simulink model "Final_Design_Updated"  (R2017b)
settings: Solver=VariableStepAuto  StartTime=0.0  StopTime=250  RelTol=1e-3
libraries: xbsIndex_r4 x101
settings Model: Creator=the20  LastModifiedBy=the20

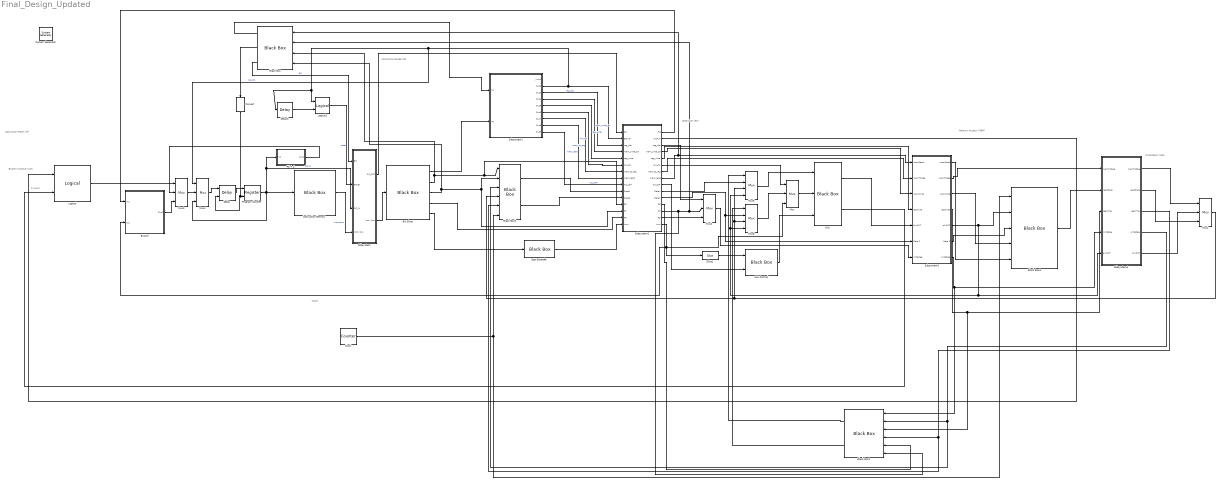
== system Final_Design_Updated ==
  note: Write Back (WB)
  note: Memory Access (MEM)
  note: Execution (EX)
  note: Instruction Dcode (ID)
  note: Branch (Control Unit)
  note: Z (ALU)
  note: Clock
  note: Instruction Fetch (IF)
  " System Generator" : xbsIndex_r4/ System Generator  Tag=genX  xilinxfamily=kintex7  part=xc7k325t  speed=-3  package=fbg676  synthesis_tool=Vivado  clock_wrapper=Clock Enables  directory=./netlist  proj_type=Vivado  Synth_file=Vivado Synthesis Defaults  Impl_file=Vivado Implementation Defaults  testbench=off  simulink_period=1  sysclk_period=10  dcm_input_clock_period=10  incr_netlist=off  trim_vbits=Everywhere in SubSystem  dbl_ovrd=According to Block Masks  core_generation=According to Block Masks  run_coregen=off  deprecated_control=off  eval_field=0  block_type=sysgen
  ALU : xbsIndex_r4/Black Box  init_code=mipsalu_config  sim_method=ISE Simulator  verbose=off  block_type=blackbox2
  ALU Control : xbsIndex_r4/Black Box  init_code=ALU_Control_config  sim_method=ISE Simulator  verbose=off  block_type=blackbox2
  Bit Slicer : xbsIndex_r4/Black Box  init_code=Bit_Slicer_config  sim_method=ISE Simulator  verbose=off  block_type=blackbox2
  Black Box : xbsIndex_r4/Black Box  init_code=Hazard_Unit_config  sim_method=ISE Simulator  verbose=off  block_type=blackbox2
  Black Box1 : xbsIndex_r4/Black Box  init_code=Forwarding_Unit_config  sim_method=ISE Simulator  verbose=off  block_type=blackbox2
  Black Box2 : xbsIndex_r4/Black Box  init_code=regFile_config  sim_method=ISE Simulator  verbose=off  block_type=blackbox2
  Black Box3 : xbsIndex_r4/Black Box  init_code=Data_Memory_config  sim_method=ISE Simulator  verbose=off  block_type=blackbox2
  Branch : Subsystem
  Clock : xbsIndex_r4/Counter  cnt_type=Free Running  cnt_to=Inf  operation=Up  start_count=0  cnt_by_val=1  arith_type=Unsigned  n_bits=1  bin_pt=0  load_pin=off  rst=off  en=off  explicit_period=on  period=1  use_behavioral_HDL=off  implementation=Fabric  dbl_ovrd=off  block_type=counter
  Convert : xbsIndex_r4/Convert  gui_display_data_type=Boolean  arith_type=Boolean  n_bits=16  bin_pt=14  float_type=Single  exp_bits=8  fraction_bits=24  quantization=Truncate  overflow=Wrap  en=off  latency=0  pipeline=off  dbl_ovrd=off  block_type=convert
  "Delay " : xbsIndex_r4/Delay  rst=off  infoeditControl=Selection of Reset will increase slice count due to use of real FFs and instead of SRLs  en=on  latency=1  reg_retiming=off  dbl_ovrd=off  block_type=delay
  Delay3 : xbsIndex_r4/Delay  rst=off  infoeditControl=Selection of Reset will increase slice count due to use of real FFs and instead of SRLs  en=off  latency=1  reg_retiming=off  dbl_ovrd=off  block_type=delay
  Instruction Memory : xbsIndex_r4/Black Box  init_code=InstructionMemory_config  sim_method=ISE Simulator  verbose=off  block_type=blackbox2
  Logical : xbsIndex_r4/Logical  logical_function=AND  inputs=2  en=off  latency=0  precision=Full  arith_type=Unsigned  n_bits=16  bin_pt=0  align_bp=on  dbl_ovrd=off  block_type=logical
  Logical1 : xbsIndex_r4/Logical  logical_function=OR  inputs=2  en=off  latency=1  precision=Full  arith_type=Unsigned  n_bits=16  bin_pt=0  align_bp=on  dbl_ovrd=off  block_type=logical
  Mux : xbsIndex_r4/Mux  inputs=2  en=off  latency=0  precision=Full  arith_type=Unsigned  n_bits=16  bin_pt=14  quantization=Truncate  overflow=Wrap  dbl_ovrd=off  block_type=mux
  Mux1 : xbsIndex_r4/Mux  inputs=2  en=off  latency=0  precision=Full  arith_type=Unsigned  n_bits=16  bin_pt=14  quantization=Truncate  overflow=Wrap  dbl_ovrd=off  block_type=mux
  Mux2 : xbsIndex_r4/Mux  inputs=2  en=off  latency=0  precision=Full  arith_type=Unsigned  n_bits=16  bin_pt=14  quantization=Truncate  overflow=Wrap  dbl_ovrd=off  block_type=mux
  Mux3 : xbsIndex_r4/Mux  inputs=2  en=off  latency=0  precision=User Defined  arith_type=Unsigned  n_bits=32  bin_pt=0  quantization=Truncate  overflow=Wrap  dbl_ovrd=off  block_type=mux
  Mux4 : xbsIndex_r4/Mux  inputs=2  en=off  latency=0  precision=User Defined  arith_type=Unsigned  n_bits=32  bin_pt=0  quantization=Truncate  overflow=Wrap  dbl_ovrd=off  block_type=mux
  Mux5 : xbsIndex_r4/Mux  inputs=3  en=off  latency=0  precision=Full  arith_type=Unsigned  n_bits=16  bin_pt=14  quantization=Truncate  overflow=Wrap  dbl_ovrd=off  block_type=mux
  Mux6 : xbsIndex_r4/Mux  inputs=3  en=off  latency=0  precision=Full  arith_type=Unsigned  n_bits=16  bin_pt=14  quantization=Truncate  overflow=Wrap  dbl_ovrd=off  block_type=mux
  PC + 4 : Subsystem
  "Program Counter " : xbsIndex_r4/Register  init=0  rst=off  en=on  dbl_ovrd=off  block_type=register
  Sign Extender : xbsIndex_r4/Black Box  init_code=Sign_Extender_config  sim_method=ISE Simulator  verbose=off  block_type=blackbox2
  Slice1 : xbsIndex_r4/Slice  nbits=6  boolean_output=off  mode=Lower Bit Location + Width  bit1=0  base1=MSB of Input  bit0=0  base0=LSB of Input  dbl_ovrd=off  block_type=slice
  Subsystem : Subsystem
  Subsystem1 : Subsystem
  Subsystem2 : Subsystem
  Subsystem3 : Subsystem
  Subsystem4 : Subsystem
  wires:
  Bit Slicer/5 -> Sign Extender/1
  Mux/1 -> ALU/2
  Mux1/1 -> Black Box2/4, Mux5/3, Mux6/3
  ALU Control/1 -> ALU/3
  Clock/1 -> Black Box3/1, Black Box2/6
  Logical/1 -> Mux3/1
  ALU/2 -> Logical/2
  "Program Counter "/1 -> PC + 4/1(In1), Subsystem/3("PC_IN "), Mux4/3, Instruction Memory/1  "PC_IN"
  Branch/1(Out1) -> Mux3/3
  PC + 4/1(Out1) -> Mux3/2
  Mux3/1 -> Mux4/2
  "Delay "/1 -> "Program Counter "/1
  Mux4/1 -> "Delay "/1
  Delay3/1 -> Logical1/2
  Black Box/2 -> Convert/1
  Black Box/3 -> Subsystem/1(EN)  "EN"
  Logical1/1 -> Subsystem/2("Reset ")  "reset"
  Instruction Memory/1 -> Subsystem/4("Instruction ")  "Instruction"
  Subsystem/2(Instruction) -> Bit Slicer/1
  Subsystem1/2(Out2) -> Subsystem2/2(Branch), Mux4/1, Delay3/1, Logical1/1  "branch"
  Bit Slicer/1 -> Subsystem1/2(In2)
  Convert/1 -> "Delay "/2, "Program Counter "/2
  Black Box/1 -> Subsystem1/1(In1)
  Subsystem/1(PC_OUT) -> Subsystem2/1("PC ")
  Subsystem2/2(branch) -> Logical/1
  Subsystem1/3(Out3) -> Subsystem2/3(reg_dst)  "reg_dst"
  Subsystem1/4(Out4) -> Subsystem2/4(mem_write_en)  "mem_write_en"
  Subsystem1/5(Out5) -> Subsystem2/5(reg_write)  "reg_write"
  Subsystem1/6(Out6) -> Subsystem2/6(Alu_src)  "Alu_src"
  Subsystem1/7(Out7) -> Subsystem2/7(mem_to_reg)  "mem_to_reg"
  Subsystem1/8(Out8) -> Subsystem2/8(mem_read)  "mem_read"
  Subsystem1/9(Out9) -> Subsystem2/9(ALU_OP)  "ALU_OP"
  Black Box2/1 -> Subsystem2/10(Data1)
  Black Box2/2 -> Subsystem2/11(Data2)
  Bit Slicer/4 -> Subsystem2/14(RD)
  Sign Extender/1 -> Subsystem2/15(Imm)
  Bit Slicer/2 -> Black Box/3, Black Box2/1, Subsystem2/12(RS)
  Bit Slicer/3 -> Black Box/4, Black Box2/2, Subsystem2/13(RT)
  Subsystem2/1(PC) -> Branch/1(In1)
  Subsystem2/3("reg_dst ") -> Mux2/1
  Subsystem2/14("RD ") -> Mux2/3
  Subsystem2/6("Alu_src ") -> Mux/1
  Subsystem2/9("ALU_OP ") -> ALU Control/2
  Mux5/1 -> ALU/1
  Mux6/1 -> Mux/2
  Subsystem2/10("Data1 ") -> Mux5/2
  Subsystem2/11("Data2 ") -> Subsystem3/6(Data 2), Mux6/2
  Subsystem2/8("mem_read ") -> Black Box/1, Subsystem3/1("memRead ")
  Subsystem2/7("mem_to_reg ") -> Subsystem3/2(memToReg)
  Subsystem2/4("mem_write_en ") -> Subsystem3/3(memWrite)
  Subsystem2/5("reg_write ") -> Subsystem3/4(regWrite)
  ALU/1 -> Subsystem3/5(aluOUT)
  Mux2/1 -> Subsystem3/7(writeReg)
  Subsystem3/1("memRead ") -> Black Box3/5
  Subsystem3/2("memToReg ") -> Subsystem4/1("memToReg ")
  Black Box3/1 -> Subsystem4/2(readData)
  Subsystem3/4("regWrite ") -> Black Box1/3, Subsystem4/3(regWrite)
  Subsystem3/7("writeReg ") -> Black Box1/1, Subsystem4/4(writeReg)
  Subsystem3/5("aluOUT ") -> Black Box3/2, Mux5/4, Mux6/4, Subsystem4/5(aluOUT)
  Subsystem3/6("Data 2 ") -> Black Box3/3
  Subsystem3/3("memWrite ") -> Black Box3/4
  Subsystem4/1("memToReg ") -> Mux1/1
  Subsystem4/2("readData ") -> Mux1/3
  Subsystem4/5("aluOUT ") -> Mux1/2
  Subsystem4/3("regWrite ") -> Black Box1/4, Black Box2/5
  Subsystem4/4("writeReg ") -> Black Box1/2, Black Box2/3
  Slice1/1 -> ALU Control/1
  Subsystem2/15("Imm ") -> Branch/2(In2), Mux/3, Slice1/1
  Black Box1/1 -> Mux5/1
  Black Box1/2 -> Mux6/1
  Subsystem2/12("RS ") -> Black Box1/5
  Subsystem2/13("RT ") -> Black Box1/6, Black Box/2, Mux2/2

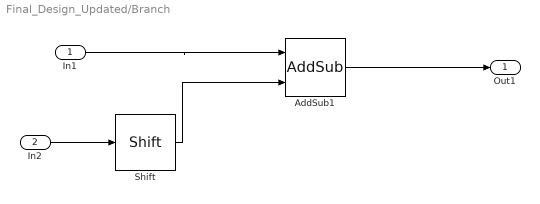
== system Final_Design_Updated/Branch ==
  In1 : Inport
  In2 : Inport  Port=2
  AddSub1 : xbsIndex_r4/AddSub  mode=Addition  use_carryin=off  use_carryout=off  en=off  latency=0  precision=User Defined  arith_type="Signed  (2's comp)"  n_bits=32  bin_pt=0  quantization=Truncate  overflow=Wrap  use_behavioral_HDL=off  hw_selection=Fabric  pipelined=off  dbl_ovrd=off  block_type=addsub
  Shift : xbsIndex_r4/Shift  shift_dir=Left  shift_bits=2  en=off  latency=0  precision=User Defined  arith_type=Unsigned  n_bits=32  bin_pt=0  quantization=Truncate  overflow=Wrap  dbl_ovrd=off  block_type=shift
  Out1 : Outport
  wires:
  AddSub1/1 -> Out1/1
  Shift/1 -> AddSub1/2
  In2/1 -> Shift/1
  In1/1 -> AddSub1/1

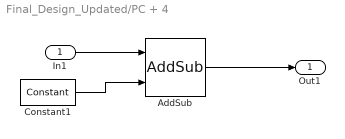
== system Final_Design_Updated/PC + 4 ==
  In1 : Inport
  AddSub : xbsIndex_r4/AddSub  mode=Addition  use_carryin=off  use_carryout=off  en=off  latency=0  precision=User Defined  arith_type=Unsigned  n_bits=32  bin_pt=0  quantization=Truncate  overflow=Wrap  use_behavioral_HDL=off  hw_selection=Fabric  pipelined=off  dbl_ovrd=off  block_type=addsub
  Constant1 : xbsIndex_r4/Constant  const=4  gui_display_data_type=Fixed-point  arith_type=Unsigned  n_bits=32  bin_pt=0  preci_type=Single  exp_width=8  frac_width=24  explicit_period=on  period=1  equ=P=C  opselect=C  inp2=PCIN>>17  opr=+  inp1=P  carry=CIN  dbl_ovrd=off  block_type=constant
  Out1 : Outport
  wires:
  Constant1/1 -> AddSub/2
  AddSub/1 -> Out1/1
  In1/1 -> AddSub/1

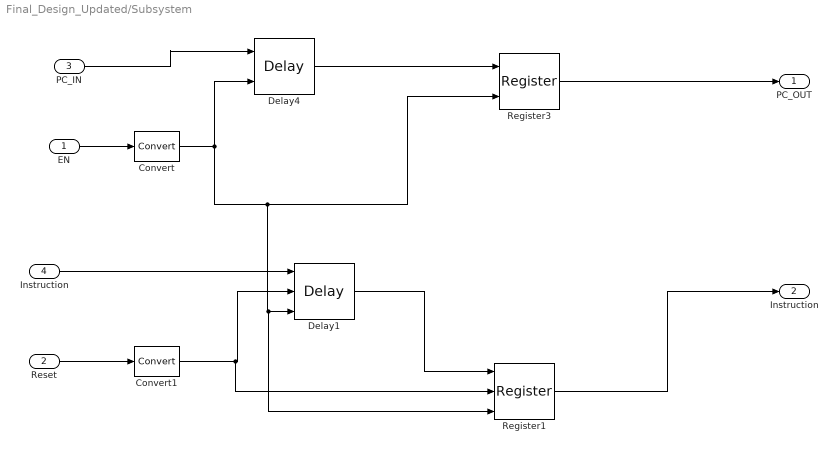
== system Final_Design_Updated/Subsystem ==
  EN : Inport
  "Reset " : Inport  Port=2
  "PC_IN " : Inport  Port=3
  "Instruction " : Inport  Port=4
  Convert : xbsIndex_r4/Convert  gui_display_data_type=Boolean  arith_type=Boolean  n_bits=16  bin_pt=0  float_type=Single  exp_bits=8  fraction_bits=24  quantization=Truncate  overflow=Wrap  en=off  latency=0  pipeline=off  dbl_ovrd=off  block_type=convert
  Convert1 : xbsIndex_r4/Convert  gui_display_data_type=Boolean  arith_type=Boolean  n_bits=16  bin_pt=0  float_type=Single  exp_bits=8  fraction_bits=24  quantization=Truncate  overflow=Wrap  en=off  latency=0  pipeline=off  dbl_ovrd=off  block_type=convert
  Delay1 : xbsIndex_r4/Delay  rst=on  infoeditControl=Selection of Reset will increase slice count due to use of real FFs and instead of SRLs  en=on  latency=1  reg_retiming=off  dbl_ovrd=off  block_type=delay
  Delay4 : xbsIndex_r4/Delay  rst=off  infoeditControl=Selection of Reset will increase slice count due to use of real FFs and instead of SRLs  en=on  latency=1  reg_retiming=off  dbl_ovrd=off  block_type=delay
  Register1 : xbsIndex_r4/Register  init=0  rst=on  en=on  dbl_ovrd=off  block_type=register
  Register3 : xbsIndex_r4/Register  init=0  rst=off  en=on  dbl_ovrd=off  block_type=register
  PC_OUT : Outport
  Instruction : Outport  Port=2
  wires:
  Delay4/1 -> Register3/1
  Delay1/1 -> Register1/1
  "PC_IN "/1 -> Delay4/1
  EN/1 -> Convert/1
  Convert/1 -> Register1/3, Delay1/3, Register3/2, Delay4/2
  Register3/1 -> PC_OUT/1
  Register1/1 -> Instruction/1
  "Reset "/1 -> Convert1/1
  Convert1/1 -> Register1/2, Delay1/2
  "Instruction "/1 -> Delay1/1

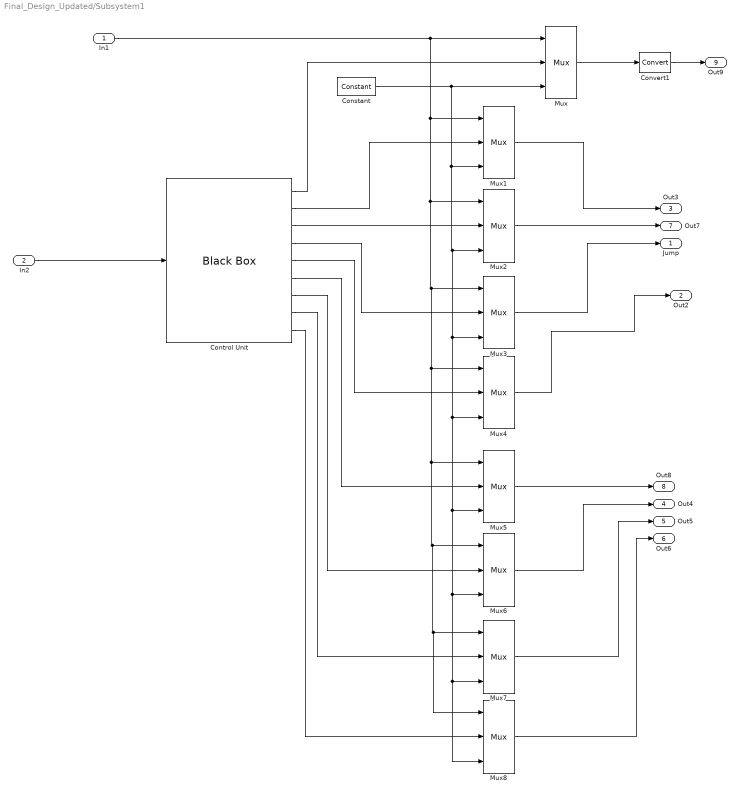
== system Final_Design_Updated/Subsystem1 ==
  In1 : Inport
  In2 : Inport  Port=2
  Constant : xbsIndex_r4/Constant  const=0  gui_display_data_type=Fixed-point  arith_type=Unsigned  n_bits=1  bin_pt=0  preci_type=Single  exp_width=8  frac_width=24  explicit_period=on  period=1  equ=P=C  opselect=C  inp2=PCIN>>17  opr=+  inp1=P  carry=CIN  dbl_ovrd=off  block_type=constant
  Control Unit : xbsIndex_r4/Black Box  init_code=Control_Unit_config  sim_method=ISE Simulator  verbose=off  block_type=blackbox2
  Convert1 : xbsIndex_r4/Convert  gui_display_data_type=Fixed-point  arith_type=Unsigned  n_bits=2  bin_pt=0  float_type=Single  exp_bits=8  fraction_bits=24  quantization=Truncate  overflow=Wrap  en=off  latency=0  pipeline=off  dbl_ovrd=off  block_type=convert
  Mux{,1..8} (9 alike) : xbsIndex_r4/Mux  inputs=2  en=off  latency=0  precision=Full  arith_type=Unsigned  n_bits=16  bin_pt=14  quantization=Truncate  overflow=Wrap  dbl_ovrd=off  block_type=mux
  Jump : Outport
  Out2 : Outport  Port=2
  Out3 : Outport  Port=3
  Out4 : Outport  Port=4
  Out5 : Outport  Port=5
  Out6 : Outport  Port=6
  Out7 : Outport  Port=7
  Out8 : Outport  Port=8
  Out9 : Outport  Port=9
  wires:
  In2/1 -> Control Unit/1
  In1/1 -> Mux1/1, Mux8/1, Mux7/1, Mux6/1, Mux5/1, Mux4/1, Mux3/1, Mux2/1, Mux/1
  Mux/1 -> Convert1/1
  Control Unit/1 -> Mux/2
  Mux1/1 -> Out3/1
  Mux2/1 -> Out7/1
  Mux3/1 -> Jump/1
  Mux4/1 -> Out2/1
  Control Unit/2 -> Mux1/2
  Control Unit/3 -> Mux2/2
  Control Unit/4 -> Mux3/2
  Control Unit/5 -> Mux4/2
  Mux5/1 -> Out8/1
  Mux6/1 -> Out4/1
  Mux7/1 -> Out5/1
  Mux8/1 -> Out6/1
  Control Unit/6 -> Mux5/2
  Control Unit/7 -> Mux6/2
  Control Unit/8 -> Mux7/2
  Control Unit/9 -> Mux8/2
  Constant/1 -> Mux/3, Mux8/3, Mux7/3, Mux6/3, Mux5/3, Mux4/3, Mux3/3, Mux2/3, Mux1/3
  Convert1/1 -> Out9/1

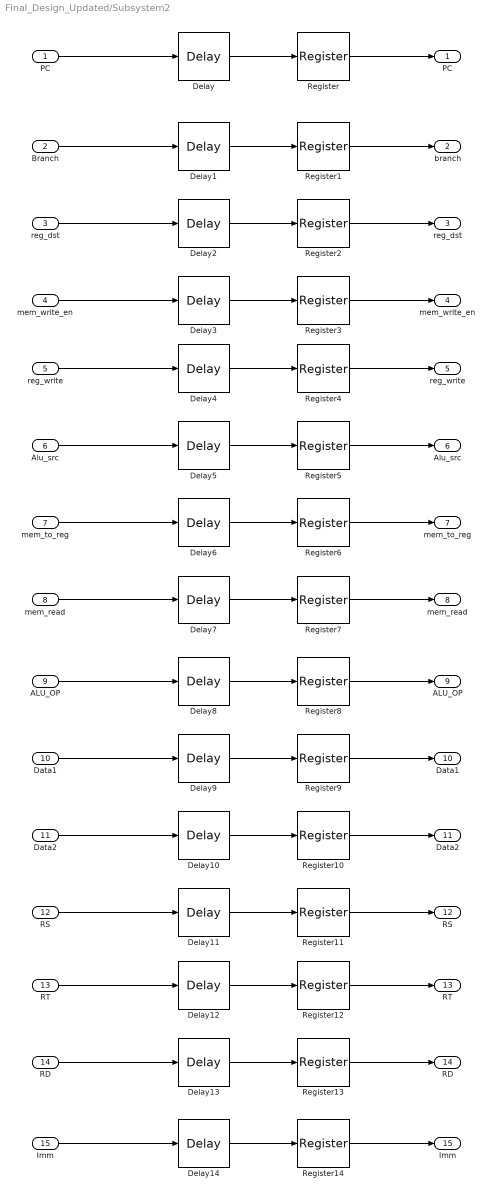
== system Final_Design_Updated/Subsystem2 ==
  "PC " : Inport
  Branch : Inport  Port=2
  reg_dst : Inport  Port=3
  mem_write_en : Inport  Port=4
  reg_write : Inport  Port=5
  Alu_src : Inport  Port=6
  mem_to_reg : Inport  Port=7
  mem_read : Inport  Port=8
  ALU_OP : Inport  Port=9
  Data1 : Inport  Port=10
  Data2 : Inport  Port=11
  RS : Inport  Port=12
  RT : Inport  Port=13
  RD : Inport  Port=14
  Imm : Inport  Port=15
  Delay{,1..14} (15 alike) : xbsIndex_r4/Delay  rst=off  infoeditControl=Selection of Reset will increase slice count due to use of real FFs and instead of SRLs  en=off  latency=1  reg_retiming=off  dbl_ovrd=off  block_type=delay
  Register{,1..14} (15 alike) : xbsIndex_r4/Register  init=0  rst=off  en=off  dbl_ovrd=off  block_type=register
  PC : Outport
  branch : Outport  Port=2
  "reg_dst " : Outport  Port=3
  "mem_write_en " : Outport  Port=4
  "reg_write " : Outport  Port=5
  "Alu_src " : Outport  Port=6
  "mem_to_reg " : Outport  Port=7
  "mem_read " : Outport  Port=8
  "ALU_OP " : Outport  Port=9
  "Data1 " : Outport  Port=10
  "Data2 " : Outport  Port=11
  "RS " : Outport  Port=12
  "RT " : Outport  Port=13
  "RD " : Outport  Port=14
  "Imm " : Outport  Port=15
  wires:
  "PC "/1 -> Delay/1
  Delay/1 -> Register/1
  Delay1/1 -> Register1/1
  Branch/1 -> Delay1/1
  Register1/1 -> branch/1
  Register/1 -> PC/1
  reg_dst/1 -> Delay2/1
  Register2/1 -> "reg_dst "/1
  Delay2/1 -> Register2/1
  mem_write_en/1 -> Delay3/1
  Register3/1 -> "mem_write_en "/1
  Delay3/1 -> Register3/1
  Alu_src/1 -> Delay5/1
  Register5/1 -> "Alu_src "/1
  mem_read/1 -> Delay7/1
  Delay7/1 -> Register7/1
  Register6/1 -> "mem_to_reg "/1
  Register7/1 -> "mem_read "/1
  Delay6/1 -> Register6/1
  mem_to_reg/1 -> Delay6/1
  Delay4/1 -> Register4/1
  Delay5/1 -> Register5/1
  Register4/1 -> "reg_write "/1
  reg_write/1 -> Delay4/1
  Data1/1 -> Delay9/1
  Register9/1 -> "Data1 "/1
  RS/1 -> Delay11/1
  Delay11/1 -> Register11/1
  Register10/1 -> "Data2 "/1
  Register11/1 -> "RS "/1
  Delay10/1 -> Register10/1
  Data2/1 -> Delay10/1
  Delay8/1 -> Register8/1
  Delay9/1 -> Register9/1
  Register8/1 -> "ALU_OP "/1
  ALU_OP/1 -> Delay8/1
  Register13/1 -> "RD "/1
  Delay13/1 -> Register13/1
  RT/1 -> Delay12/1
  RD/1 -> Delay13/1
  Register12/1 -> "RT "/1
  Delay12/1 -> Register12/1
  Delay14/1 -> Register14/1
  Register14/1 -> "Imm "/1
  Imm/1 -> Delay14/1

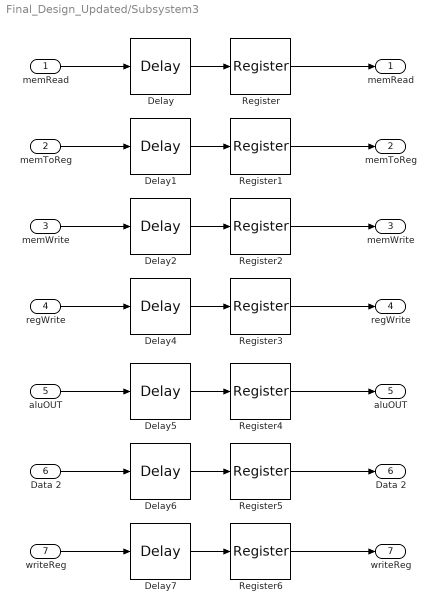
== system Final_Design_Updated/Subsystem3 ==
  "memRead " : Inport
  memToReg : Inport  Port=2
  memWrite : Inport  Port=3
  regWrite : Inport  Port=4
  aluOUT : Inport  Port=5
  Data 2 : Inport  Port=6
  writeReg : Inport  Port=7
  Delay{,1..2,4..7} (7 alike) : xbsIndex_r4/Delay  rst=off  infoeditControl=Selection of Reset will increase slice count due to use of real FFs and instead of SRLs  en=off  latency=1  reg_retiming=off  dbl_ovrd=off  block_type=delay
  Register{,1..6} (7 alike) : xbsIndex_r4/Register  init=0  rst=off  en=off  dbl_ovrd=off  block_type=register
  "memRead " : Outport
  "memToReg " : Outport  Port=2
  "memWrite " : Outport  Port=3
  "regWrite " : Outport  Port=4
  "aluOUT " : Outport  Port=5
  "Data 2 " : Outport  Port=6
  "writeReg " : Outport  Port=7
  wires:
  Delay6/1 -> Register5/1
  memWrite/1 -> Delay2/1
  Register5/1 -> "Data 2 "/1
  Register4/1 -> "aluOUT "/1
  writeReg/1 -> Delay7/1
  Register2/1 -> "memWrite "/1
  aluOUT/1 -> Delay5/1
  Delay7/1 -> Register6/1
  Delay5/1 -> Register4/1
  Delay2/1 -> Register2/1
  Data 2/1 -> Delay6/1
  Register3/1 -> "regWrite "/1
  Register/1 -> "memRead "/1
  Delay1/1 -> Register1/1
  Register6/1 -> "writeReg "/1
  Delay4/1 -> Register3/1
  memToReg/1 -> Delay1/1
  "memRead "/1 -> Delay/1
  Register1/1 -> "memToReg "/1
  Delay/1 -> Register/1
  regWrite/1 -> Delay4/1

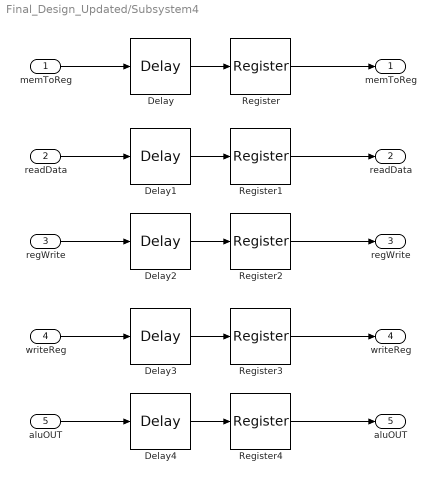
== system Final_Design_Updated/Subsystem4 ==
  "memToReg " : Inport
  readData : Inport  Port=2
  regWrite : Inport  Port=3
  writeReg : Inport  Port=4
  aluOUT : Inport  Port=5
  Delay{,1..4} (5 alike) : xbsIndex_r4/Delay  rst=off  infoeditControl=Selection of Reset will increase slice count due to use of real FFs and instead of SRLs  en=off  latency=1  reg_retiming=off  dbl_ovrd=off  block_type=delay
  Register{,1..4} (5 alike) : xbsIndex_r4/Register  init=0  rst=off  en=off  dbl_ovrd=off  block_type=register
  "memToReg " : Outport
  "readData " : Outport  Port=2
  "regWrite " : Outport  Port=3
  "writeReg " : Outport  Port=4
  "aluOUT " : Outport  Port=5
  wires:
  Register/1 -> "memToReg "/1
  "memToReg "/1 -> Delay/1
  Delay/1 -> Register/1
  readData/1 -> Delay1/1
  Delay1/1 -> Register1/1
  Register1/1 -> "readData "/1
  Delay2/1 -> Register2/1
  Register2/1 -> "regWrite "/1
  regWrite/1 -> Delay2/1
  writeReg/1 -> Delay3/1
  Register3/1 -> "writeReg "/1
  Delay3/1 -> Register3/1
  Delay4/1 -> Register4/1
  Register4/1 -> "aluOUT "/1
  aluOUT/1 -> Delay4/1
